simulink model "Copy_of_Formation_Controller"  (R2022b)
settings: Solver=VariableStepAuto  StartTime=0.0  StopTime=10.0  FixedStep=CONTROL_CONST.dt  MaxStep=0.01  RelTol=1e-3
values from neighbouring files (symbols this model uses):
  CONTROL_PARAM = Simulink.Parameter(CONTROL_PARAM_VALUE)    [control_model_init.m]
undefined symbols (not defined in the file or in its folder): actuator_cmd, CONTROL_CONST, CONTROL_PARAM_VALUE, CTRL_PARAM, DiscIntNeverNeededParam, FROMATION_PARAM, timestamp
libraries: FC_Lib x5, simulink x4, simulink_extras x1, aerolibasang x1
settings Model: VariantFading=off  Creator=19114  LastModifiedBy=19114
settings OptimizationCC: DefaultParameterBehavior=Inlined  DefaultUnderspecifiedDataType=single  EnhancedBackFolding=on  PassReuseOutputArgsAs=Individual arguments  ZeroExternalMemoryAtStartup=off  ZeroInternalMemoryAtStartup=off  OptimizeBlockOrder=speed  DifferentSizesBufferReuse=on  OptimizationCustomize=off  EfficientTunableParamExpr=on
settings DebuggingCC: ParameterTunabilityLossMsg=error
settings HardwareCC: ProdBitPerPointer=32  ProdBitPerSizeT=32  ProdBitPerPtrDiffT=32  ProdWordSize=32  ProdHWDeviceType=Intel->x86-32 (Windows32)
settings SFSimCC: MATLABDynamicMemAlloc=off
settings RTWCC: Description=Embedded Coder  SystemTargetFile=ert.tlc  TemplateMakefile=ert_default_tmf
settings CodeAppCC: ForceParamTrailComments=on  IgnoreCustomStorageClasses=off  OperatorAnnotations=on  SimulinkDataObjDesc=on  SFDataObjDesc=on  InsertBlockDesc=on
settings ERTTargetCC: TargetLangStandard=C99 (ISO)  GenerateSampleERTMain=on  SupportVariableSizeSignals=on  InlinedParameterPlacement=NonHierarchical  ERTCustomFileTemplate=example_file_process.tlc

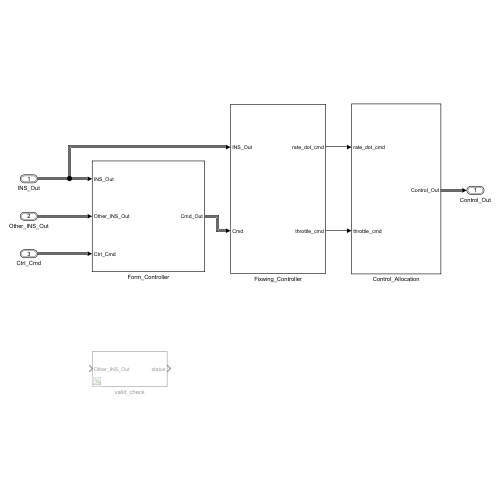
[thumbnail: Simulink's stored preview of the top-level diagram]
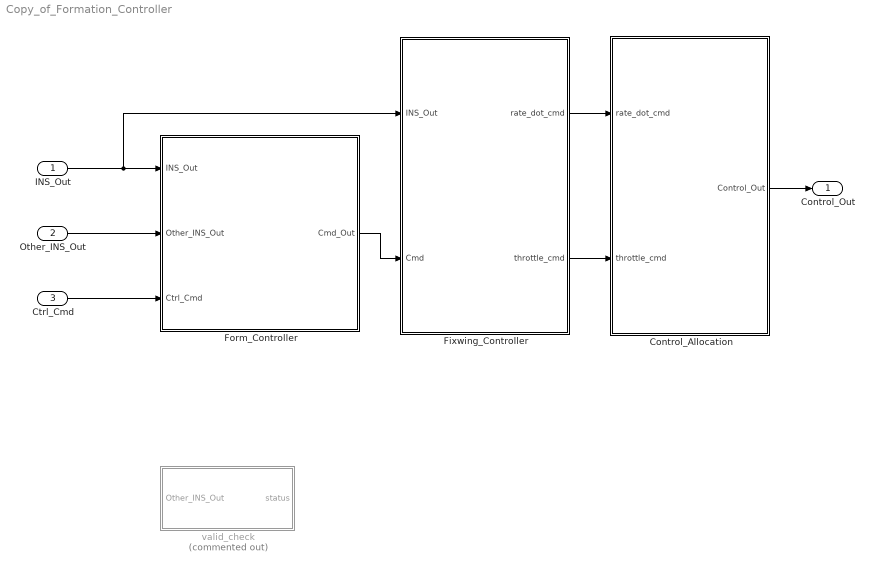
== system Copy_of_Formation_Controller ==
  INS_Out : Inport  OutDataTypeStr=Bus: INS_Out_Bus
  Other_INS_Out : Inport  Port=2  OutDataTypeStr=Bus: Other_INS_Out_Bus
  Ctrl_Cmd : Inport  Port=3  OutDataTypeStr=Bus: Cmd_In_Bus
  Control_Allocation : Subsystem
  Fixwing_Controller : Subsystem
  Form_Controller : Subsystem
  valid_check : Subsystem  Commented=on
  Control_Out : Outport  OutDataTypeStr=Bus: Control_Out_Bus
  wires:
  INS_Out/1 -> Fixwing_Controller/1(INS_Out), Form_Controller/1(INS_Out)
  Other_INS_Out/1 -> Form_Controller/2(Other_INS_Out)
  Ctrl_Cmd/1 -> Form_Controller/3(Ctrl_Cmd)
  Control_Allocation/1(Control_Out) -> Control_Out/1
  Form_Controller/1(Cmd_Out) -> Fixwing_Controller/2(Cmd)
  Fixwing_Controller/1(rate_dot_cmd) -> Control_Allocation/1(rate_dot_cmd)
  Fixwing_Controller/2(throttle_cmd) -> Control_Allocation/2(throttle_cmd)

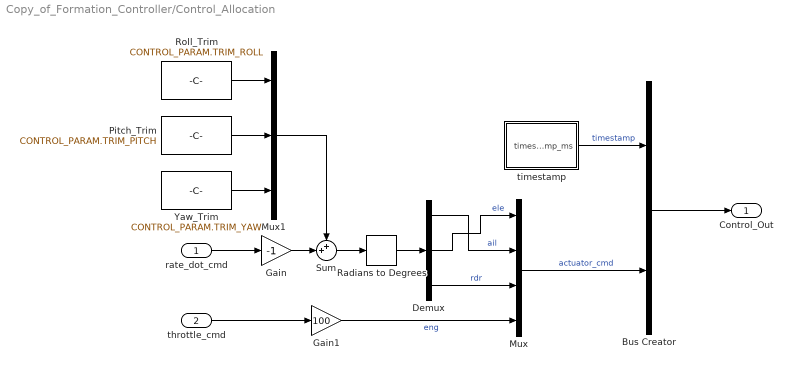
== system Copy_of_Formation_Controller/Control_Allocation ==
  rate_dot_cmd : Inport
  throttle_cmd : Inport  Port=2
  Bus Creator : BusCreator  Inputs=timestamp,actuator_cmd  OutDataTypeStr=Bus: Control_Out_Bus
  Demux : Demux  Outputs=3
  Gain : Gain  Gain=-1
  Gain1 : Gain  Gain=100
  Mux : Mux
  Mux1 : Mux  Inputs=3
  Pitch_Trim : Constant  Value=CONTROL_PARAM.TRIM_PITCH
  Radians to Degrees : simulink_extras/Transformations/Radians to Degrees
  Roll_Trim : Constant  Value=CONTROL_PARAM.TRIM_ROLL
  Sum : Sum  Inputs=++|
  Yaw_Trim : Constant  Value=CONTROL_PARAM.TRIM_YAW
  timestamp : Subsystem  mask{sample_time=CONTROL_CONST.dt*1000}
      mask prompts: sample_time "sample time (ms)"
  Control_Out : Outport
  wires:
  Bus Creator/1 -> Control_Out/1
  Mux/1 -> Bus Creator/2  "actuator_cmd"
  rate_dot_cmd/1 -> Gain/1
  throttle_cmd/1 -> Gain1/1
  Demux/1 -> Mux/2  "ail"
  Demux/2 -> Mux/1  "ele"
  Demux/3 -> Mux/3  "rdr"
  Sum/1 -> Radians to Degrees/1
  Mux1/1 -> Sum/1
  Gain/1 -> Sum/2
  Radians to Degrees/1 -> Demux/1
  Gain1/1 -> Mux/4  "eng"
  timestamp/1(timestamp_ms) -> Bus Creator/1  "timestamp"
  Roll_Trim/1 -> Mux1/1
  Pitch_Trim/1 -> Mux1/2
  Yaw_Trim/1 -> Mux1/3

== system Copy_of_Formation_Controller/Fixwing_Controller ==
  INS_Out : Inport
  Cmd : Inport  Port=2
  Attitude_Control : Subsystem
  Lateral_Longitudinal_Control : Subsystem
  rate_dot_cmd : Outport
  throttle_cmd : Outport  Port=2
  wires:
  Cmd/1 -> Lateral_Longitudinal_Control/2(Cmd)
  Attitude_Control/1(rate_dot_cmd) -> rate_dot_cmd/1
  INS_Out/1 -> Attitude_Control/1(INS_Out), Lateral_Longitudinal_Control/1(INS_Out)
  Lateral_Longitudinal_Control/2(throttle_cmd) -> throttle_cmd/1
  Lateral_Longitudinal_Control/1(att_cmd) -> Attitude_Control/2(att_cmd)

== system Copy_of_Formation_Controller/Form_Controller ==
  INS_Out : Inport
  Other_INS_Out : Inport  Port=2
  Ctrl_Cmd : Inport  Port=3
  Add : Sum
  Add1 : Sum
  Add2 : Sum
  Bus Creator : BusCreator  Inputs=3
  Consensus_Controller : Subsystem
  Local_State_Controller : Subsystem
  Cmd_Out : Outport
  wires:
  Add/1 -> Bus Creator/1  "cmd_ax"
  Local_State_Controller/1(ax_cmd) -> Add/1
  Consensus_Controller/1(ax_cmd) -> Add/2
  Add1/1 -> Bus Creator/2  "cmd_ay"
  Local_State_Controller/2(ay_cmd) -> Add1/1
  Local_State_Controller/3(vh_cmd) -> Add2/1
  Consensus_Controller/2(ay_cmd) -> Add1/2
  Add2/1 -> Bus Creator/3  "cmd_vh"
  Consensus_Controller/3(vh_cmd) -> Add2/2
  Other_INS_Out/1 -> Consensus_Controller/2(Other_INS_Out)
  Ctrl_Cmd/1 -> Local_State_Controller/1(Ctrl_Cmd)
  INS_Out/1 -> Consensus_Controller/1(INS_Out), Local_State_Controller/2(INS_Out)
  Bus Creator/1 -> Cmd_Out/1

== system Copy_of_Formation_Controller/valid_check ==
  Other_INS_Out : Inport
  Bus Selector1 : BusSelector  OutputSignals=timestamp
  Data Type Conversion : DataTypeConversion  OutDataTypeStr=uint32  SaturateOnIntegerOverflow=off  RndMeth=Floor
  Detect Increase : simulink/Logic and Bit Operations/Detect Increase  vinit=0.0  OutDataTypeStr=boolean
  Selector : Selector  InputPortWidth=20  IndexOptions=Index vector (dialog)  Indices=[1:CTRL_PARAM.NUM_UAV]  OutputSizes=1
  status : Outport
  wires:
  Other_INS_Out/1 -> Bus Selector1/1
  Detect Increase/1 -> Selector/1
  Bus Selector1/1 -> Detect Increase/1  "<timestamp>"
  Selector/1 -> Data Type Conversion/1
  Data Type Conversion/1 -> status/1  "status"

== system Copy_of_Formation_Controller/Control_Allocation/timestamp ==
  Add : Sum
  Constant : Constant  Value=sample_time  OutDataTypeStr=uint32
  Memory : Memory
  timestamp_ms : Outport  VectorParamsAs1DForOutWhenUnconnected=off
  wires:
  Constant/1 -> Add/1
  Add/1 -> Memory/1, timestamp_ms/1
  Memory/1 -> Add/2

== system Copy_of_Formation_Controller/Fixwing_Controller/Attitude_Control ==
  INS_Out : Inport
  att_cmd : Inport  Port=2
  Innerloop_Rate_Control : Subsystem
  Outloop_Angle_Control : Subsystem
  rate_dot_cmd : Outport  VectorParamsAs1DForOutWhenUnconnected=off
  wires:
  Outloop_Angle_Control/1(euler_rate_cmd) -> Innerloop_Rate_Control/1(euler_rate_cmd)
  INS_Out/1 -> Innerloop_Rate_Control/2(INS_Out), Outloop_Angle_Control/2(INS_Out)
  Innerloop_Rate_Control/1(rate_dot_cmd) -> rate_dot_cmd/1
  att_cmd/1 -> Outloop_Angle_Control/1(att_cmd)

== system Copy_of_Formation_Controller/Fixwing_Controller/Lateral_Longitudinal_Control ==
  INS_Out : Inport
  Cmd : Inport  Port=2
  Airspeed_Filter : Subsystem
  Altitude_Control : Subsystem
  Lateral_Control : Subsystem
  Longitudinal_Control : Subsystem
  Mux : Mux  Inputs=2
  att_cmd : Outport  VectorParamsAs1DForOutWhenUnconnected=off
  throttle_cmd : Outport  Port=2  VectorParamsAs1DForOutWhenUnconnected=off
  wires:
  Cmd/1 -> Lateral_Control/1(Cmd), Airspeed_Filter/1(Cmd), Altitude_Control/1(Cmd)
  Altitude_Control/1(alt_rate_sp) -> Longitudinal_Control/1(alt_rate_sp)
  INS_Out/1 -> Longitudinal_Control/4(INS_Out), Airspeed_Filter/2(INS_Out), Altitude_Control/2(INS_Out)
  Longitudinal_Control/1(pitch_cmd) -> Mux/2  "pitch_cmd"
  Altitude_Control/2(alt_rate) -> Longitudinal_Control/2(alt_rate)
  Longitudinal_Control/2(throttle_cmd) -> throttle_cmd/1
  Airspeed_Filter/1(airspeed) -> Longitudinal_Control/3(airspeed)
  Lateral_Control/1(roll_cmd) -> Mux/1  "roll_cmd"
  Mux/1 -> att_cmd/1

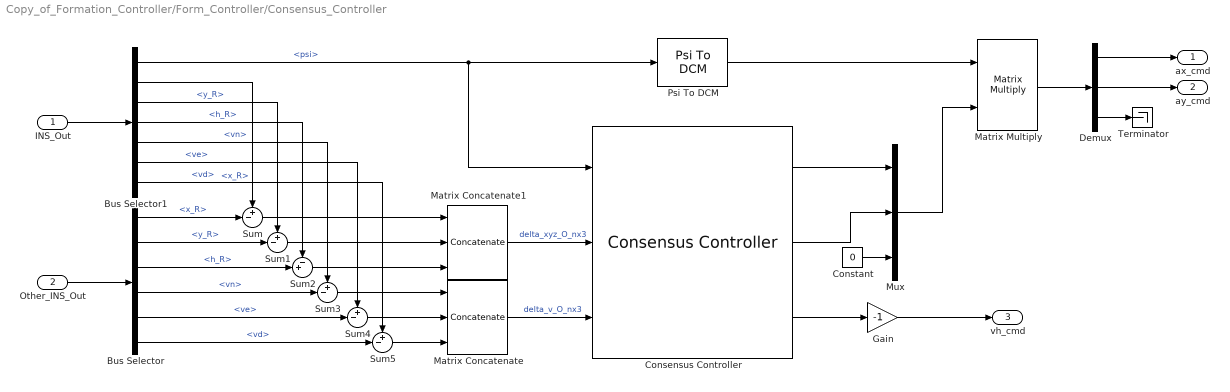
== system Copy_of_Formation_Controller/Form_Controller/Consensus_Controller ==
  INS_Out : Inport
  Other_INS_Out : Inport  Port=2
  Bus Selector : BusSelector  OutputSignals=x_R,y_R,h_R,vn,ve,vd
  Bus Selector1 : BusSelector  OutputSignals=psi,x_R,y_R,h_R,vn,ve,vd
  Consensus Controller : FC_Lib/Fromation/Consensus Controller  uav_id=FROMATION_PARAM.UAV_ID+1  adj_matrix=FROMATION_PARAM.ADJ_MARTIX  rel_x=FROMATION_PARAM.REL_X_MATRIX  rel_y=FROMATION_PARAM.REL_Y_MATRIX  rel_z=FROMATION_PARAM.REL_Z_MATRIX  kx=FROMATION_PARAM.FORM_X_KP  ky=FROMATION_PARAM.FORM_Y_KP  kz=FROMATION_PARAM.FORM_Z_KP
      settings: LibrarySourceBlock=|
      | simulink/User-Defined
      | Functions/MATLAB Function
  Constant : Constant  Value=0  OutDataTypeStr=single
  Demux : Demux  Outputs=3
  Gain : Gain  Gain=-1
  Matrix Concatenate : Concatenate  NumInputs=3  Mode=Multidimensional array  ConcatenateDimension=2
  Matrix Concatenate1 : Concatenate  NumInputs=3  Mode=Multidimensional array  ConcatenateDimension=2
  Matrix Multiply : Product  Multiplication=Matrix(*)
  Mux : Mux  Inputs=3
  Psi To DCM : FC_Lib/Transformation/Psi To DCM
      settings: SourceProductName=Flight Control Toolbox
  Sum{,1,3..5} (5 alike) : Sum  Inputs=+-|
  Sum2 : Sum  Inputs=-+|
  Terminator : Terminator
  ax_cmd : Outport
  ay_cmd : Outport  Port=2
  vh_cmd : Outport  Port=3
  wires:
  Bus Selector1/4 -> Sum2/1  "<h_R>"
  Bus Selector/6 -> Sum5/2  "<vd>"
  Other_INS_Out/1 -> Bus Selector/1
  Bus Selector/2 -> Sum1/2  "<y_R>"
  Sum2/1 -> Matrix Concatenate1/3
  INS_Out/1 -> Bus Selector1/1
  Bus Selector/5 -> Sum4/2  "<ve>"
  Bus Selector1/7 -> Sum5/1  "<vd>"
  Bus Selector1/6 -> Sum4/1  "<ve>"
  Bus Selector1/2 -> Sum/1  "<x_R>"
  Bus Selector/3 -> Sum2/2  "<h_R>"
  Bus Selector/1 -> Sum/2  "<x_R>"
  Bus Selector/4 -> Sum3/2  "<vn>"
  Sum4/1 -> Matrix Concatenate/2
  Sum1/1 -> Matrix Concatenate1/2
  Bus Selector1/5 -> Sum3/1  "<vn>"
  Sum5/1 -> Matrix Concatenate/3
  Matrix Concatenate/1 -> Consensus Controller/3  "delta_v_O_nx3"
  Sum/1 -> Matrix Concatenate1/1
  Matrix Concatenate1/1 -> Consensus Controller/2  "delta_xyz_O_nx3"
  Bus Selector1/3 -> Sum1/1  "<y_R>"
  Consensus Controller/3 -> Gain/1
  Sum3/1 -> Matrix Concatenate/1
  Consensus Controller/2 -> Mux/2
  Consensus Controller/1 -> Mux/1
  Gain/1 -> vh_cmd/1
  Constant/1 -> Mux/3
  Psi To DCM/1 -> Matrix Multiply/1
  Mux/1 -> Matrix Multiply/2
  Matrix Multiply/1 -> Demux/1
  Demux/3 -> Terminator/1
  Bus Selector1/1 -> Consensus Controller/1, Psi To DCM/1  "<psi>"
  Demux/1 -> ax_cmd/1
  Demux/2 -> ay_cmd/1

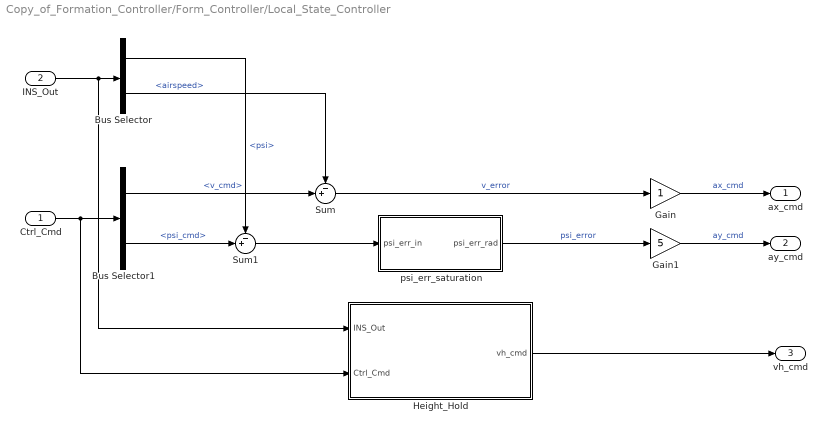
== system Copy_of_Formation_Controller/Form_Controller/Local_State_Controller ==
  Ctrl_Cmd : Inport
  INS_Out : Inport  Port=2
  Bus Selector : BusSelector  OutputSignals=psi,airspeed
  Bus Selector1 : BusSelector  OutputSignals=v_cmd,psi_cmd
  Gain : Gain
  Gain1 : Gain  Gain=5
  Height_Hold : Subsystem
  Sum : Sum  Inputs=-+|
  Sum1 : Sum  Inputs=-+|
  psi_err_saturation : Subsystem
  ax_cmd : Outport
  ay_cmd : Outport  Port=2
  vh_cmd : Outport  Port=3
  wires:
  Sum/1 -> Gain/1  "v_error"
  Sum1/1 -> psi_err_saturation/1(psi_err_in)
  Gain/1 -> ax_cmd/1  "ax_cmd"
  Gain1/1 -> ay_cmd/1  "ay_cmd"
  Bus Selector/1 -> Sum1/1  "<psi>"
  Bus Selector1/1 -> Sum/2  "<v_cmd>"
  Bus Selector1/2 -> Sum1/2  "<psi_cmd>"
  psi_err_saturation/1(psi_err_rad) -> Gain1/1  "psi_error"
  Ctrl_Cmd/1 -> Height_Hold/2(Ctrl_Cmd), Bus Selector1/1
  INS_Out/1 -> Height_Hold/1(INS_Out), Bus Selector/1
  Height_Hold/1(vh_cmd) -> vh_cmd/1
  Bus Selector/2 -> Sum/1  "<airspeed>"

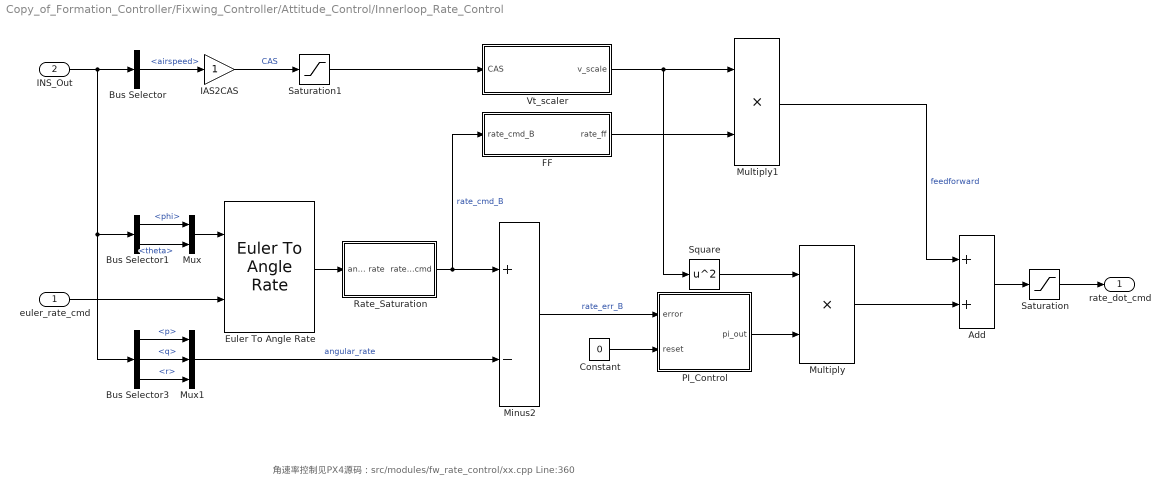
== system Copy_of_Formation_Controller/Fixwing_Controller/Attitude_Control/Innerloop_Rate_Control ==
  note: 角速率控制见PX4源码：src/modules/fw_rate_control/xx.cpp Line:360
  euler_rate_cmd : Inport
  INS_Out : Inport  Port=2
  Add : Sum
  Bus Selector : BusSelector  OutputSignals=airspeed
  Bus Selector1 : BusSelector  OutputSignals=phi,theta
  Bus Selector3 : BusSelector  OutputSignals=p,q,r
  Constant : Constant  Value=0
  Euler To Angle Rate : FC_Lib/Math/Euler To Angle Rate
      settings: SourceProductName=Flight Control Toolbox
  FF : Subsystem
  IAS2CAS : Gain
  Minus2 : Sum  Inputs=+-
  Multiply : Product
  Multiply1 : Product
  Mux : Mux  Inputs=2
  Mux1 : Mux  Inputs=3
  PI_Control : Subsystem
  Rate_Saturation : Subsystem
  Saturation : Saturate  UpperLimit=1  LowerLimit=-1
  Saturation1 : Saturate  UpperLimit=inf  LowerLimit=0.5
  Square : Math  Operator=square
  Vt_scaler : Subsystem
  rate_dot_cmd : Outport  VectorParamsAs1DForOutWhenUnconnected=off
  wires:
  Vt_scaler/1(v_scale) -> Square/1, Multiply1/1
  FF/1(rate_ff) -> Multiply1/2
  Multiply1/1 -> Add/1  "feedforward"
  Bus Selector/1 -> IAS2CAS/1  "<airspeed>"
  euler_rate_cmd/1 -> Euler To Angle Rate/2
  Euler To Angle Rate/1 -> Rate_Saturation/1(angle rate)
  Mux1/1 -> Minus2/2  "angular_rate"
  Add/1 -> Saturation/1
  Minus2/1 -> PI_Control/1(error)  "rate_err_B"
  PI_Control/1(pi_out) -> Multiply/2
  INS_Out/1 -> Bus Selector/1, Bus Selector3/1, Bus Selector1/1
  Bus Selector1/1 -> Mux/1  "<phi>"
  Bus Selector1/2 -> Mux/2  "<theta>"
  Mux/1 -> Euler To Angle Rate/1
  Bus Selector3/1 -> Mux1/1  "<p>"
  Bus Selector3/2 -> Mux1/2  "<q>"
  Bus Selector3/3 -> Mux1/3  "<r>"
  Saturation1/1 -> Vt_scaler/1(CAS)
  IAS2CAS/1 -> Saturation1/1  "CAS"
  Square/1 -> Multiply/1
  Saturation/1 -> rate_dot_cmd/1
  Constant/1 -> PI_Control/2(reset)
  Multiply/1 -> Add/2
  Rate_Saturation/1(rate_cmd) -> FF/1(rate_cmd_B), Minus2/1  "rate_cmd_B"

== system Copy_of_Formation_Controller/Fixwing_Controller/Attitude_Control/Outloop_Angle_Control ==
  att_cmd : Inport
  INS_Out : Inport  Port=2
  Attitude_Controller : Subsystem
  Heading_Controller : Subsystem
  Mux : Mux  Inputs=2
  Reshape : Reshape  OutputDimensionality=Column vector (2-D)
  euler_rate_cmd : Outport  VectorParamsAs1DForOutWhenUnconnected=off
  wires:
  INS_Out/1 -> Heading_Controller/2(INS_Out), Attitude_Controller/2(INS_Out)
  Attitude_Controller/1(phi_theta_rate_cmd) -> Mux/1
  Heading_Controller/1(psi_rate_cmd) -> Mux/2
  Mux/1 -> Reshape/1
  Reshape/1 -> euler_rate_cmd/1
  att_cmd/1 -> Heading_Controller/1(att_cmd), Attitude_Controller/1(att_cmd)

== system Copy_of_Formation_Controller/Fixwing_Controller/Lateral_Longitudinal_Control/Airspeed_Filter ==
  Cmd : Inport
  INS_Out : Inport  Port=2
  Bus Creator : BusCreator  Inputs=3
  Bus Selector1 : BusSelector  OutputSignals=airspeed
  Calc_TAS_Rate_Setpoint : Subsystem
  Constant : Constant  Value=0  OutDataTypeStr=single
  Ideal Airspeed Correction : aerolibasang/Ideal Airspeed Correction  Commented=on  units=Metric (MKS)  vel_in=CAS  vel_out_tas=CAS  vel_out_eas=TAS  vel_out_cas=TAS  method=Table Lookup  SubOnly=on  action=None
  Saturation2 : Saturate  UpperLimit=inf  LowerLimit=0
  Second Order DT Filter : FC_Lib/Filter/Second Order DT Filter  fc=10  zeta=1
      settings: SourceProductName=Flight Control Toolbox
  airspeed : Outport
  wires:
  INS_Out/1 -> Bus Selector1/1
  Bus Creator/1 -> airspeed/1
  Bus Selector1/1 -> Second Order DT Filter/1, Saturation2/1, Calc_TAS_Rate_Setpoint/2(TAS_mPs)  "<airspeed>"
  Cmd/1 -> Calc_TAS_Rate_Setpoint/1(Cmd)
  Calc_TAS_Rate_Setpoint/1(TAS_rate_sp_mPs) -> Bus Creator/1  "TAS_rate_sp_mPs"
  Saturation2/1 -> Bus Creator/2  "TAS_mPs"
  Second Order DT Filter/1 -> Bus Creator/3  "TAS_rate_mPs"
  Constant/1 -> Second Order DT Filter/2

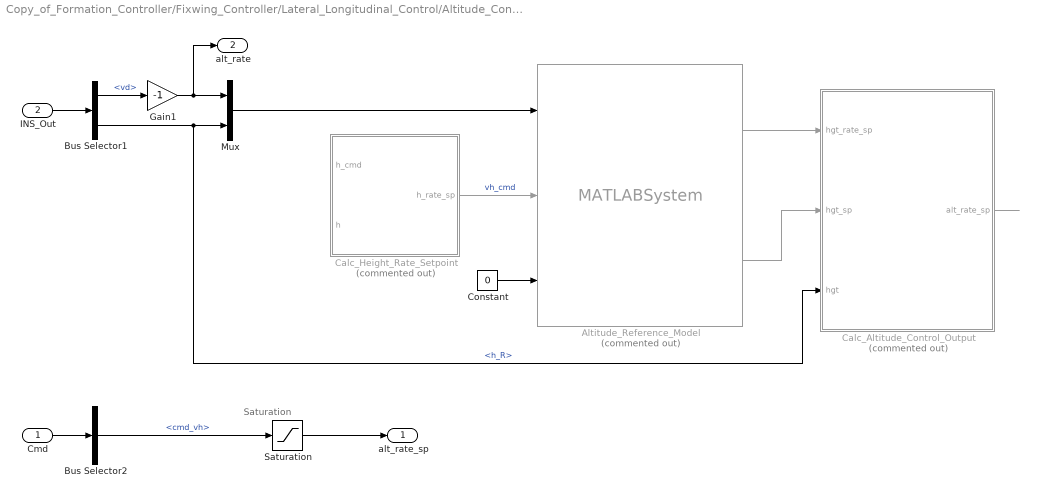
== system Copy_of_Formation_Controller/Fixwing_Controller/Lateral_Longitudinal_Control/Altitude_Control ==
  note: Saturation
  Cmd : Inport
  INS_Out : Inport  Port=2
  Altitude_Reference_Model : MATLABSystem  Commented=on  System=VelocitySmoothing  max_jerk=single(1000)  max_accel=CONTROL_PARAM.FW_T_VERT_ACC  max_climb_rate=CONTROL_PARAM.FW_T_CLMB_MAX  max_sink_rate=CONTROL_PARAM.FW_T_SINK_MAX  SampleTime=CONTROL_CONST.dt  SimulateUsing=Code generation
      mask Type: VelocitySmoothing
      mask Display:
      | disp(['Velocity' char(10) 'Smoothing']);
      | port_label('input',1,'v0x0');
      | port_label('input',2,'vel_sp');
      | port_label('input',3,'reset');
      | port_label('output',1,'vel');
      | port_label('output',2,'pos');
  Bus Selector1 : BusSelector  OutputSignals=vd,h_R
  Bus Selector2 : BusSelector  OutputSignals=cmd_vh
  Calc_Altitude_Control_Output : Subsystem  Commented=on
  Calc_Height_Rate_Setpoint : Subsystem  Commented=on
  Constant : Constant  Value=0  OutDataTypeStr=single
  Gain1 : Gain  Gain=-1
  Mux : Mux  Inputs=2
  Saturation : Saturate  UpperLimit=CONTROL_PARAM.FW_T_CLMB_MAX  LowerLimit=-CONTROL_PARAM.FW_T_SINK_MAX
  alt_rate_sp : Outport
  alt_rate : Outport  Port=2
  wires:
  Cmd/1 -> Bus Selector2/1
  INS_Out/1 -> Bus Selector1/1
  Bus Selector1/2 -> Mux/2, Calc_Altitude_Control_Output/3(hgt)  "<h_R>"
  Bus Selector2/1 -> Saturation/1  "<cmd_vh>"
  Bus Selector1/1 -> Gain1/1  "<vd>"
  Gain1/1 -> Mux/1, alt_rate/1
  Mux/1 -> Altitude_Reference_Model/1
  Altitude_Reference_Model/2 -> Calc_Altitude_Control_Output/2(hgt_sp)
  Constant/1 -> Altitude_Reference_Model/3
  Altitude_Reference_Model/1 -> Calc_Altitude_Control_Output/1(hgt_rate_sp)
  Calc_Altitude_Control_Output/1(alt_rate_sp) -> ?
  Calc_Height_Rate_Setpoint/1(h_rate_sp) -> Altitude_Reference_Model/2  "vh_cmd"
  Saturation/1 -> alt_rate_sp/1

== system Copy_of_Formation_Controller/Fixwing_Controller/Lateral_Longitudinal_Control/Lateral_Control ==
  Cmd : Inport
  Atan : Trigonometry  Operator=atan
  Bus Selector : BusSelector  OutputSignals=cmd_ay
  Constant : Constant  Value=CONTROL_CONST.g
  Product : Product  Inputs=/*
  Saturation : Saturate  UpperLimit=CONTROL_PARAM.FW_R_LIM  LowerLimit=-CONTROL_PARAM.FW_R_LIM
  roll_cmd : Outport
  wires:
  Cmd/1 -> Bus Selector/1
  Constant/1 -> Product/1
  Bus Selector/1 -> Product/2  "<cmd_ay>"
  Product/1 -> Atan/1
  Atan/1 -> Saturation/1
  Saturation/1 -> roll_cmd/1

== system Copy_of_Formation_Controller/Fixwing_Controller/Lateral_Longitudinal_Control/Longitudinal_Control ==
  alt_rate_sp : Inport
  alt_rate : Inport  Port=2
  airspeed : Inport  Port=3
  INS_Out : Inport  Port=4
  Bus Selector : BusSelector  OutputSignals=TAS_mPs
  Calc_Specific_Energy_Rates : Subsystem
  Pitch_Control : Subsystem
  Throttle_Control : Subsystem
  pitch_cmd : Outport
  throttle_cmd : Outport  Port=2
  wires:
  alt_rate_sp/1 -> Calc_Specific_Energy_Rates/1(alt_rate_sp)
  alt_rate/1 -> Calc_Specific_Energy_Rates/2(alt_rate)
  Throttle_Control/1(throttle_cmd) -> throttle_cmd/1
  Pitch_Control/1(pitch_cmd) -> pitch_cmd/1
  INS_Out/1 -> Throttle_Control/2(INS_Out)
  Calc_Specific_Energy_Rates/1(ser) -> Pitch_Control/1(ser), Throttle_Control/1(ser)
  Bus Selector/1 -> Pitch_Control/2(tas)  "<TAS_mPs>"
  airspeed/1 -> Bus Selector/1, Calc_Specific_Energy_Rates/3(airspeed)

== system Copy_of_Formation_Controller/Form_Controller/Local_State_Controller/Height_Hold ==
  INS_Out : Inport
  Ctrl_Cmd : Inport  Port=2
  Bus Selector2 : BusSelector  OutputSignals=h_cmd
  Bus Selector3 : BusSelector  OutputSignals=h_R
  Gain3 : Gain
  Sum3 : Sum  Inputs=-+|
  vh_cmd : Outport
  wires:
  Bus Selector3/1 -> Sum3/1  "<h_R>"
  Sum3/1 -> Gain3/1  "h_error"
  INS_Out/1 -> Bus Selector3/1
  Bus Selector2/1 -> Sum3/2  "<h_cmd>"
  Ctrl_Cmd/1 -> Bus Selector2/1
  Gain3/1 -> vh_cmd/1

== system Copy_of_Formation_Controller/Form_Controller/Local_State_Controller/psi_err_saturation ==
  psi_err_in : Inport
  Abs : Abs  SaturateOnIntegerOverflow=off
  Compare To Constant : simulink/Logic and Bit Operations/Compare To Constant  relop=>  const=pi  OutDataTypeStr=boolean
  Constant : Constant  Value=2*pi  OutDataTypeStr=single
  Multiply : Product
  Sign : Signum
  Subtract : Sum  Inputs=-+
  Switch : Switch  Criteria=u2 > Threshold  SaturateOnIntegerOverflow=off  InputSameDT=off
  psi_err_rad : Outport  VectorParamsAs1DForOutWhenUnconnected=off
  wires:
  Multiply/1 -> Switch/1
  Sign/1 -> Multiply/2
  Subtract/1 -> Multiply/1
  Constant/1 -> Subtract/1
  Switch/1 -> psi_err_rad/1
  Compare To Constant/1 -> Switch/2
  Abs/1 -> Compare To Constant/1, Subtract/2
  psi_err_in/1 -> Abs/1, Switch/3, Sign/1

== system Copy_of_Formation_Controller/Fixwing_Controller/Attitude_Control/Innerloop_Rate_Control/FF ==
  rate_cmd_B : Inport
  Demux : Demux  Outputs=3
  Mux2 : Mux  Inputs=3
  pitch_ff : Gain  Gain=CONTROL_PARAM.FW_PR_FF
  roll_ff : Gain  Gain=CONTROL_PARAM.FW_RR_FF
  yaw_ff : Gain  Gain=CONTROL_PARAM.FW_YR_FF
  rate_ff : Outport
  wires:
  Mux2/1 -> rate_ff/1
  Demux/2 -> pitch_ff/1  "pitch_rate"
  Demux/1 -> roll_ff/1  "roll_rate"
  Demux/3 -> yaw_ff/1  "yaw_rate"
  rate_cmd_B/1 -> Demux/1
  roll_ff/1 -> Mux2/1
  pitch_ff/1 -> Mux2/2
  yaw_ff/1 -> Mux2/3

== system Copy_of_Formation_Controller/Fixwing_Controller/Attitude_Control/Innerloop_Rate_Control/PI_Control ==
  error : Inport
  reset : Inport  Port=2
  Add1 : Sum
  I_Control : Subsystem  mask{p_ki=CONTROL_PARAM.ROLL_RATE_I, q_ki=CONTROL_PARAM.PITCH_RATE_I, r_ki=CONTROL_PARAM.YAW_RATE_I, max_i=CONTROL_PARAM.RATE_I_MAX, min_i=CONTROL_PARAM.RATE_I_MIN}
  P_Control : Subsystem  mask{p_kp=CONTROL_PARAM.ROLL_RATE_P, q_kp=CONTROL_PARAM.PITCH_RATE_P, r_kp=CONTROL_PARAM.YAW_RATE_P}
  pi_out : Outport  VectorParamsAs1DForOutWhenUnconnected=off
  wires:
  Add1/1 -> pi_out/1
  I_Control/1(i_out) -> Add1/2  "i_out"
  error/1 -> P_Control/1(err), I_Control/1(err)
  P_Control/1(p_out) -> Add1/1
  reset/1 -> I_Control/2(reset)

== system Copy_of_Formation_Controller/Fixwing_Controller/Attitude_Control/Innerloop_Rate_Control/Rate_Saturation ==
  angle rate : Inport
  Demux : Demux  Outputs=3
  Mux : Mux  Inputs=3
  Saturation : Saturate  UpperLimit=CONTROL_PARAM.FW_R_RMAX  LowerLimit=-CONTROL_PARAM.FW_R_RMAX
  Saturation1 : Saturate  UpperLimit=CONTROL_PARAM.FW_P_RMAX  LowerLimit=-CONTROL_PARAM.FW_P_RMAX
  Saturation2 : Saturate  UpperLimit=CONTROL_PARAM.FW_Y_RMAX  LowerLimit=-CONTROL_PARAM.FW_Y_RMAX
  rate_cmd : Outport
  wires:
  angle rate/1 -> Demux/1
  Mux/1 -> rate_cmd/1
  Demux/1 -> Saturation/1  "roll_rate"
  Demux/2 -> Saturation1/1  "pitch_rate"
  Demux/3 -> Saturation2/1  "yaw_rate"
  Saturation/1 -> Mux/1
  Saturation1/1 -> Mux/2
  Saturation2/1 -> Mux/3

== system Copy_of_Formation_Controller/Fixwing_Controller/Attitude_Control/Innerloop_Rate_Control/Vt_scaler ==
  CAS : Inport
  CAS_constrained : Saturate  UpperLimit=CONTROL_PARAM.FW_AIRSPD_MAX  LowerLimit=CONTROL_PARAM.FW_AIRSPD_STALL
  Constant1 : Constant  Value=CONTROL_PARAM.FW_ARSP_SCALE_EN
  Constant2 : Constant  OutDataTypeStr=single
  Divide : Product  Inputs=/*
  Switch1 : Switch  Criteria=u2 > Threshold  SaturateOnIntegerOverflow=off  InputSameDT=off
  Trim_CAS : Constant  Value=CONTROL_PARAM.FW_AIRSPD_TRIM
  v_scale : Outport
  wires:
  CAS_constrained/1 -> Divide/1
  Divide/1 -> Switch1/1
  Constant1/1 -> Switch1/2
  Switch1/1 -> v_scale/1
  Trim_CAS/1 -> Divide/2
  Constant2/1 -> Switch1/3
  CAS/1 -> CAS_constrained/1

== system Copy_of_Formation_Controller/Fixwing_Controller/Attitude_Control/Outloop_Angle_Control/Attitude_Controller ==
  att_cmd : Inport
  INS_Out : Inport  Port=2
  Error : Subsystem
  P_Controller : Subsystem
  phi_theta_rate_cmd : Outport  VectorParamsAs1DForOutWhenUnconnected=off
  wires:
  INS_Out/1 -> Error/2(INS_Out)
  P_Controller/1(u) -> phi_theta_rate_cmd/1
  att_cmd/1 -> Error/1(att_cmd)
  Error/1(euler_err_rad) -> P_Controller/1(error)

== system Copy_of_Formation_Controller/Fixwing_Controller/Attitude_Control/Outloop_Angle_Control/Heading_Controller ==
  att_cmd : Inport
  INS_Out : Inport  Port=2
  Selector : Selector  InputPortWidth=2  IndexOptions=Index vector (dialog)  Indices=[1]  OutputSizes=1
  Turning_Coordination : Subsystem
  psi_rate_cmd : Outport  VectorParamsAs1DForOutWhenUnconnected=off
  wires:
  Turning_Coordination/1(psi_rate_sp) -> psi_rate_cmd/1
  INS_Out/1 -> Turning_Coordination/2(INS_Out)
  att_cmd/1 -> Selector/1
  Selector/1 -> Turning_Coordination/1(phi_sp)

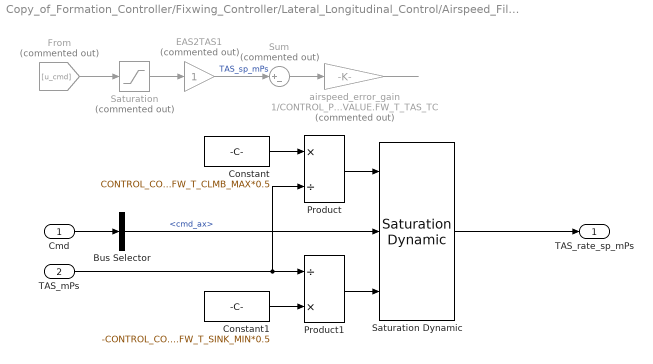
== system Copy_of_Formation_Controller/Fixwing_Controller/Lateral_Longitudinal_Control/Airspeed_Filter/Calc_TAS_Rate_Setpoint ==
  Cmd : Inport
  TAS_mPs : Inport  Port=2
  Bus Selector : BusSelector  OutputSignals=cmd_ax
  Constant : Constant  Value=CONTROL_CONST.g*CONTROL_PARAM.FW_T_CLMB_MAX*0.5  OutDataTypeStr=single
  Constant1 : Constant  Value=-CONTROL_CONST.g*CONTROL_PARAM.FW_T_SINK_MIN*0.5  OutDataTypeStr=single
  EAS2TAS1 : Gain  Commented=on
  From : From  Commented=on  GotoTag=u_cmd
  Product : Product  Inputs=*/
  Product1 : Product  Inputs=/*
  Saturation : Saturate  Commented=on  UpperLimit=CONTROL_PARAM.FW_AIRSPD_MAX  LowerLimit=CONTROL_PARAM.FW_AIRSPD_MIN
  Saturation Dynamic : simulink/Discontinuities/Saturation Dynamic  OutMin=[]  OutMax=[]  OutDataTypeStr=Inherit: Same as second input  OutDataType=fixdt(1, 16)  OutScaling=2^-10  DoSatur=off
  Sum : Sum  Commented=on  Inputs=|+-
  airspeed_error_gain : Gain  Commented=on  Gain=1/CONTROL_PARAM_VALUE.FW_T_TAS_TC
  TAS_rate_sp_mPs : Outport
  wires:
  Saturation Dynamic/1 -> TAS_rate_sp_mPs/1
  Sum/1 -> airspeed_error_gain/1
  Cmd/1 -> Bus Selector/1
  TAS_mPs/1 -> Product/2, Product1/1
  airspeed_error_gain/1 -> ?
  Constant/1 -> Product/1
  Product/1 -> Saturation Dynamic/1
  Product1/1 -> Saturation Dynamic/3
  Constant1/1 -> Product1/2
  From/1 -> Saturation/1
  EAS2TAS1/1 -> Sum/1  "TAS_sp_mPs"
  Saturation/1 -> EAS2TAS1/1
  Bus Selector/1 -> Saturation Dynamic/2  "<cmd_ax>"

== system Copy_of_Formation_Controller/Fixwing_Controller/Lateral_Longitudinal_Control/Altitude_Control/Calc_Altitude_Control_Output ==
  note: Saturation
  hgt_rate_sp : Inport
  hgt_sp : Inport  Port=2
  hgt : Inport  Port=3
  Gain : Gain  Gain=CONTROL_PARAM.FW_T_HRATE_FF
  Gain2 : Gain  Gain=1/max(CONTROL_PARAM.FW_T_ALT_TC,0.1)
  Saturation : Saturate  UpperLimit=CONTROL_PARAM.FW_T_CLMB_MAX  LowerLimit=-CONTROL_PARAM.FW_T_SINK_MAX
  Sum : Sum  Inputs=|++
  Sum1 : Sum  Inputs=|+-
  alt_rate_sp : Outport
  wires:
  Sum1/1 -> Gain2/1
  hgt_sp/1 -> Sum1/1
  Gain/1 -> Sum/1  "alt_rate_gain_ff"
  hgt_rate_sp/1 -> Gain/1
  hgt/1 -> Sum1/2
  Sum/1 -> Saturation/1
  Gain2/1 -> Sum/2  "alt_gain"
  Saturation/1 -> alt_rate_sp/1

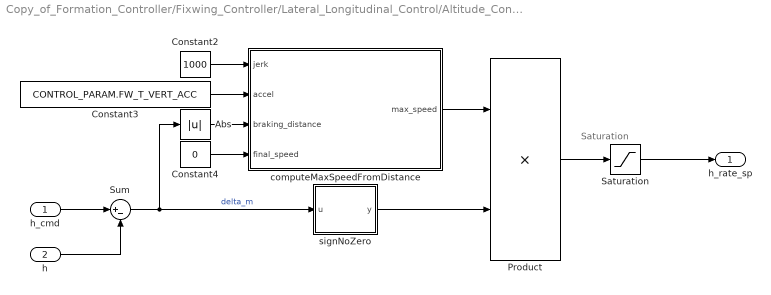
== system Copy_of_Formation_Controller/Fixwing_Controller/Lateral_Longitudinal_Control/Altitude_Control/Calc_Height_Rate_Setpoint ==
  note: Saturation
  h_cmd : Inport
  h : Inport  Port=2
  Abs : Abs  SaturateOnIntegerOverflow=off
  Constant2 : Constant  Value=1000  OutDataTypeStr=single
  Constant3 : Constant  Value=CONTROL_PARAM.FW_T_VERT_ACC  OutDataTypeStr=single
  Constant4 : Constant  Value=0  OutDataTypeStr=single
  Product : Product
  Saturation : Saturate  UpperLimit=min(CONTROL_PARAM.FW_T_CLMB_R_SP, CONTROL_PARAM.FW_T_CLMB_MAX)  LowerLimit=-min(CONTROL_PARAM.FW_T_SINK_R_SP, CONTROL_PARAM.FW_T_SINK_MAX)
  Sum : Sum  Inputs=|+-  OutDataTypeStr=Inherit: Same as first input
  computeMaxSpeedFromDistance : MATLAB Function  TreatAsAtomicUnit=on
  signNoZero : MATLAB Function  TreatAsAtomicUnit=on
  h_rate_sp : Outport  OutDataTypeStr=single
  wires:
  computeMaxSpeedFromDistance/1(max_speed) -> Product/1
  Constant3/1 -> computeMaxSpeedFromDistance/2(accel)
  h/1 -> Sum/2
  Sum/1 -> Abs/1, signNoZero/1(u)  "delta_m"
  Abs/1 -> computeMaxSpeedFromDistance/3(braking_distance)
  Constant2/1 -> computeMaxSpeedFromDistance/1(jerk)
  Constant4/1 -> computeMaxSpeedFromDistance/4(final_speed)
  signNoZero/1(y) -> Product/2
  h_cmd/1 -> Sum/1
  Product/1 -> Saturation/1
  Saturation/1 -> h_rate_sp/1

== system Copy_of_Formation_Controller/Fixwing_Controller/Lateral_Longitudinal_Control/Longitudinal_Control/Calc_Specific_Energy_Rates ==
  alt_rate_sp : Inport
  alt_rate : Inport  Port=2
  airspeed : Inport  Port=3
  Bus Creator : BusCreator  Inputs=4
  Bus Selector : BusSelector  OutputSignals=TAS_mPs,TAS_rate_sp_mPs,TAS_rate_mPs
  Constant : Constant  Value=CONTROL_CONST.g
  Product{1..4} (4 alike) : Product
  ser : Outport
  wires:
  Product4/1 -> Bus Creator/1  "spe_rate_sp"
  airspeed/1 -> Bus Selector/1
  Bus Selector/1 -> Product3/2, Product1/1  "<TAS_mPs>"
  Bus Selector/2 -> Product1/2  "<TAS_rate_sp_mPs>"
  Product1/1 -> Bus Creator/3  "ske_rate_sp"
  Bus Selector/3 -> Product3/1  "<TAS_rate_mPs>"
  Product2/1 -> Bus Creator/2  "spe_rate"
  Product3/1 -> Bus Creator/4  "ske_rate"
  Bus Creator/1 -> ser/1
  Constant/1 -> Product4/2, Product2/1
  alt_rate/1 -> Product2/2
  alt_rate_sp/1 -> Product4/1

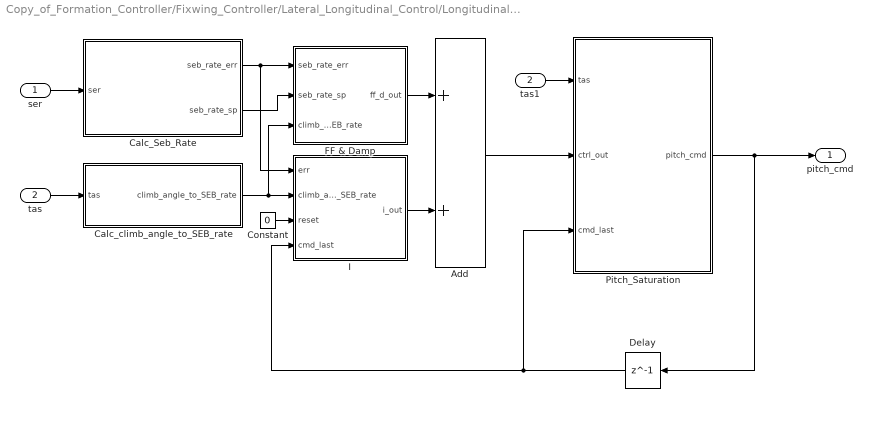
== system Copy_of_Formation_Controller/Fixwing_Controller/Lateral_Longitudinal_Control/Longitudinal_Control/Pitch_Control ==
  ser : Inport
  tas : Inport  Port=2
  Add : Sum
  Calc_Seb_Rate : Subsystem
  Calc_climb_angle_to_SEB_rate : Subsystem
  Constant : Constant  Value=0  OutDataTypeStr=single
  Delay : Delay  DelayLength=1
  FF & Damp : Subsystem
  I : Subsystem
  Pitch_Saturation : Subsystem
  tas1 : InportShadow  Port=2
  pitch_cmd : Outport
  wires:
  ser/1 -> Calc_Seb_Rate/1(ser)
  Calc_Seb_Rate/1(seb_rate_err) -> I/1(err), FF & Damp/1(seb_rate_err)
  I/1(i_out) -> Add/2
  Delay/1 -> I/4(cmd_last), Pitch_Saturation/3(cmd_last)
  Calc_Seb_Rate/2(seb_rate_sp) -> FF & Damp/2(seb_rate_sp)
  FF & Damp/1(ff_d_out) -> Add/1
  Pitch_Saturation/1(pitch_cmd) -> pitch_cmd/1, Delay/1
  Add/1 -> Pitch_Saturation/2(ctrl_out)
  Constant/1 -> I/3(reset)
  tas/1 -> Calc_climb_angle_to_SEB_rate/1(tas)
  Calc_climb_angle_to_SEB_rate/1(climb_angle_to_SEB_rate) -> FF & Damp/3(climb_angle_to_SEB_rate), I/2(climb_angle_to_SEB_rate)
  tas1/1 -> Pitch_Saturation/1(tas)

== system Copy_of_Formation_Controller/Fixwing_Controller/Lateral_Longitudinal_Control/Longitudinal_Control/Throttle_Control ==
  note: limit
  ser : Inport
  INS_Out : Inport  Port=2
  Add : Sum
  Calc_STE_Rate : Subsystem
  Constant : Constant  Value=0  OutDataTypeStr=single
  Damp : Subsystem
  Delay : Delay  DelayLength=1
  I : Subsystem
  Saturation : Saturate  UpperLimit=CONTROL_PARAM.FW_THR_MAX  LowerLimit=CONTROL_PARAM.FW_THR_MIN
  throttle_cmd : Outport
  wires:
  ser/1 -> Calc_STE_Rate/1(ser)
  I/1(i_out) -> Add/2
  Delay/1 -> I/3(cmd_last)
  Add/1 -> Saturation/1
  Calc_STE_Rate/2(throttle_predicted) -> Damp/2(throttle_predicted)
  Saturation/1 -> throttle_cmd/1, Delay/1
  Calc_STE_Rate/1(ste_rate_err) -> Damp/1(ste_rate_err), I/1(ste_rate_err)
  Damp/1(ff_d_out) -> Add/1
  Constant/1 -> I/2(reset)
  INS_Out/1 -> Calc_STE_Rate/2(INS_Out)

== system Copy_of_Formation_Controller/Fixwing_Controller/Attitude_Control/Innerloop_Rate_Control/PI_Control/I_Control ==
  err : Inport
  reset : Inport  Port=2
  Constant : Constant  Value=[0;0;0]  OutDataTypeStr=single
  Discrete-Time Integrator : DiscreteIntegrator  ExternalReset=level  InitialConditionSource=external  SampleTime=-1  LimitOutput=on  UpperSaturationLimit=max_i  LowerSaturationLimit=min_i  ICPrevOutput=DiscIntNeverNeededParam  ICPrevScaledInput=DiscIntNeverNeededParam
  Multiply : Product  OutDataTypeStr=Inherit: Same as first input
  Mux : Mux  Inputs=3
  gain1 : Constant  Value=p_ki  OutDataTypeStr=single
  gain2 : Constant  Value=q_ki  OutDataTypeStr=single
  gain3 : Constant  Value=r_ki  OutDataTypeStr=single
  i_out : Outport  VectorParamsAs1DForOutWhenUnconnected=off
  wires:
  err/1 -> Multiply/2
  gain2/1 -> Mux/2
  gain1/1 -> Mux/1
  gain3/1 -> Mux/3
  reset/1 -> Discrete-Time Integrator/2
  Constant/1 -> Discrete-Time Integrator/3
  Discrete-Time Integrator/1 -> i_out/1
  Mux/1 -> Multiply/1
  Multiply/1 -> Discrete-Time Integrator/1

== system Copy_of_Formation_Controller/Fixwing_Controller/Attitude_Control/Innerloop_Rate_Control/PI_Control/P_Control ==
  err : Inport
  Multiply : Product  OutDataTypeStr=Inherit: Same as first input
  Mux : Mux  Inputs=3
  gain1 : Constant  Value=p_kp  OutDataTypeStr=single
  gain2 : Constant  Value=q_kp  OutDataTypeStr=single
  gain3 : Constant  Value=r_kp  OutDataTypeStr=single
  p_out : Outport  VectorParamsAs1DForOutWhenUnconnected=off
  wires:
  err/1 -> Multiply/2
  gain2/1 -> Mux/2
  Mux/1 -> Multiply/1
  gain1/1 -> Mux/1
  Multiply/1 -> p_out/1
  gain3/1 -> Mux/3

== system Copy_of_Formation_Controller/Fixwing_Controller/Attitude_Control/Outloop_Angle_Control/Attitude_Controller/Error ==
  att_cmd : Inport
  INS_Out : Inport  Port=2
  Bus_Select : Subsystem
  Demux : Demux  Outputs=2
  Mux : Mux  Inputs=2
  Pitch Offset : Bias  Bias=CONTROL_PARAM.FW_PSP_OFF  SaturateOnIntegerOverflow=off
  Sum : Sum  Inputs=|+-
  euler_err_rad : Outport  VectorParamsAs1DForOutWhenUnconnected=off
  wires:
  att_cmd/1 -> Demux/1  "att_cmd_B_rad"
  Sum/1 -> euler_err_rad/1  "att_error_B_rad"
  INS_Out/1 -> Bus_Select/1(INS_Out)
  Bus_Select/1(att_est_B_rad) -> Sum/2  "att_est_B_rad"
  Demux/2 -> Pitch Offset/1
  Demux/1 -> Mux/1
  Pitch Offset/1 -> Mux/2
  Mux/1 -> Sum/1

== system Copy_of_Formation_Controller/Fixwing_Controller/Attitude_Control/Outloop_Angle_Control/Attitude_Controller/P_Controller ==
  error : Inport
  Constant1 : Constant  Value=CONTROL_PARAM.ROLL_P
  Constant2 : Constant  Value=CONTROL_PARAM.PITCH_P
  Multiply : Product
  Mux : Mux  Inputs=2
  u : Outport  VectorParamsAs1DForOutWhenUnconnected=off
  wires:
  Multiply/1 -> u/1
  error/1 -> Multiply/1
  Mux/1 -> Multiply/2
  Constant1/1 -> Mux/1
  Constant2/1 -> Mux/2

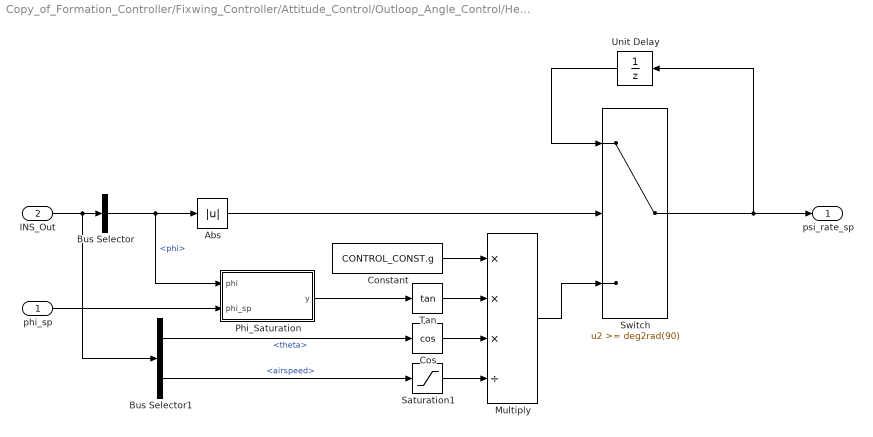
== system Copy_of_Formation_Controller/Fixwing_Controller/Attitude_Control/Outloop_Angle_Control/Heading_Controller/Turning_Coordination ==
  phi_sp : Inport
  INS_Out : Inport  Port=2
  Abs : Abs  SaturateOnIntegerOverflow=off
  Bus Selector : BusSelector  OutputSignals=phi
  Bus Selector1 : BusSelector  OutputSignals=theta,airspeed
  Constant : Constant  Value=CONTROL_CONST.g  OutDataTypeStr=single
  Cos : Trigonometry  Operator=cos
  Multiply : Product  Inputs=***/
  Phi_Saturation : Subsystem
  Saturation1 : Saturate  UpperLimit=CONTROL_PARAM.FW_AIRSPD_MAX  LowerLimit=CONTROL_PARAM.FW_AIRSPD_STALL
  Switch : Switch  Threshold=deg2rad(90)  SaturateOnIntegerOverflow=off  InputSameDT=off
  Tan : Trigonometry  Operator=tan
  Unit Delay : UnitDelay  SampleTime=-1  HasFrameUpgradeWarning=on
  psi_rate_sp : Outport  VectorParamsAs1DForOutWhenUnconnected=off
  wires:
  Tan/1 -> Multiply/2
  Cos/1 -> Multiply/3
  Bus Selector/1 -> Phi_Saturation/1(phi), Abs/1  "<phi>"
  INS_Out/1 -> Bus Selector/1, Bus Selector1/1
  Bus Selector1/1 -> Cos/1  "<theta>"
  Abs/1 -> Switch/2
  Unit Delay/1 -> Switch/1
  Multiply/1 -> Switch/3
  Switch/1 -> Unit Delay/1, psi_rate_sp/1
  Constant/1 -> Multiply/1
  Saturation1/1 -> Multiply/4
  Bus Selector1/2 -> Saturation1/1  "<airspeed>"
  phi_sp/1 -> Phi_Saturation/2(phi_sp)
  Phi_Saturation/1(y) -> Tan/1

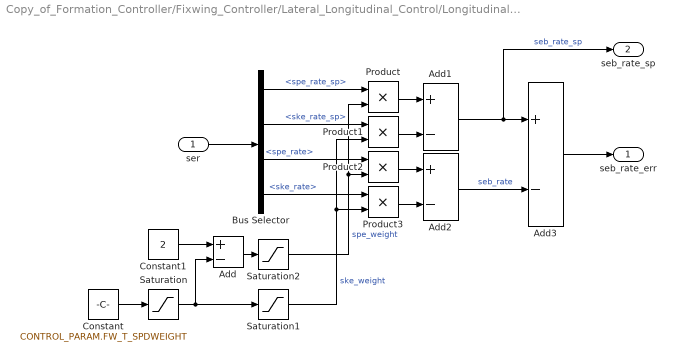
== system Copy_of_Formation_Controller/Fixwing_Controller/Lateral_Longitudinal_Control/Longitudinal_Control/Pitch_Control/Calc_Seb_Rate ==
  ser : Inport
  Add{,1..3} (4 alike) : Sum  Inputs=+-
  Bus Selector : BusSelector  OutputSignals=spe_rate_sp,ske_rate_sp,spe_rate,ske_rate
  Constant : Constant  Value=CONTROL_PARAM.FW_T_SPDWEIGHT  OutDataTypeStr=single
  Constant1 : Constant  Value=2  OutDataTypeStr=single
  Product{,1..3} (4 alike) : Product
  Saturation : Saturate  UpperLimit=2  LowerLimit=0
  Saturation1 : Saturate  UpperLimit=1  LowerLimit=0
  Saturation2 : Saturate  UpperLimit=1  LowerLimit=0
  seb_rate_err : Outport
  seb_rate_sp : Outport  Port=2
  wires:
  Saturation2/1 -> Product2/2, Product/2  "spe_weight"
  Add/1 -> Saturation2/1
  Saturation/1 -> Add/2, Saturation1/1
  Saturation1/1 -> Product1/2, Product3/2  "ske_weight"
  Constant1/1 -> Add/1
  Constant/1 -> Saturation/1
  ser/1 -> Bus Selector/1
  Bus Selector/1 -> Product/1  "<spe_rate_sp>"
  Bus Selector/2 -> Product1/1  "<ske_rate_sp>"
  Bus Selector/3 -> Product2/1  "<spe_rate>"
  Bus Selector/4 -> Product3/1  "<ske_rate>"
  Product1/1 -> Add1/2
  Product/1 -> Add1/1
  Product2/1 -> Add2/1
  Product3/1 -> Add2/2
  Add1/1 -> seb_rate_sp/1, Add3/1  "seb_rate_sp"
  Add2/1 -> Add3/2  "seb_rate"
  Add3/1 -> seb_rate_err/1

== system Copy_of_Formation_Controller/Fixwing_Controller/Lateral_Longitudinal_Control/Longitudinal_Control/Pitch_Control/Calc_climb_angle_to_SEB_rate ==
  tas : Inport
  Constant1 : Constant  Value=CONTROL_CONST.g
  Product : Product
  climb_angle_to_SEB_rate : Outport
  wires:
  Constant1/1 -> Product/1
  Product/1 -> climb_angle_to_SEB_rate/1
  tas/1 -> Product/2

== system Copy_of_Formation_Controller/Fixwing_Controller/Lateral_Longitudinal_Control/Longitudinal_Control/Pitch_Control/FF & Damp ==
  seb_rate_err : Inport
  seb_rate_sp : Inport  Port=2
  climb_angle_to_SEB_rate : Inport  Port=3
  Add : Sum
  Divide : Product  Inputs=*/
  pitch_damping_gain : Gain  Gain=CONTROL_PARAM.FW_T_PTCH_DAMP
  seb_rate_ff : Gain  Gain=CONTROL_PARAM.FW_T_SEB_R_FF
  ff_d_out : Outport
  wires:
  seb_rate_err/1 -> pitch_damping_gain/1
  seb_rate_sp/1 -> seb_rate_ff/1
  pitch_damping_gain/1 -> Add/1
  seb_rate_ff/1 -> Add/2
  Add/1 -> Divide/1
  climb_angle_to_SEB_rate/1 -> Divide/2
  Divide/1 -> ff_d_out/1

== system Copy_of_Formation_Controller/Fixwing_Controller/Lateral_Longitudinal_Control/Longitudinal_Control/Pitch_Control/I ==
  err : Inport
  climb_angle_to_SEB_rate : Inport  Port=2
  reset : Inport  Port=3
  cmd_last : Inport  Port=4
  Discrete-Time Integrator : DiscreteIntegrator  gainval=1  ExternalReset=level  SampleTime=-1  ICPrevOutput=DiscIntNeverNeededParam  ICPrevScaledInput=DiscIntNeverNeededParam
  Divide : Product  Inputs=*/
  Error_Saturation : MATLAB Function  TreatAsAtomicUnit=on  mask{uplimit=CONTROL_PARAM.FW_P_LIM_MAX, downlimit=CONTROL_PARAM.FW_P_LIM_MIN}
      mask prompts: uplimit "MaxOutput"; downlimit "MinOutput"
  I_Gain : Gain  Gain=CONTROL_PARAM.FW_T_I_GAIN_PIT
  i_out : Outport
  wires:
  Discrete-Time Integrator/1 -> i_out/1
  err/1 -> Divide/1
  cmd_last/1 -> Error_Saturation/2(cmd_last)
  Error_Saturation/1(y) -> I_Gain/1
  reset/1 -> Discrete-Time Integrator/2
  climb_angle_to_SEB_rate/1 -> Divide/2
  Divide/1 -> Error_Saturation/1(err)
  I_Gain/1 -> Discrete-Time Integrator/1

== system Copy_of_Formation_Controller/Fixwing_Controller/Lateral_Longitudinal_Control/Longitudinal_Control/Pitch_Control/Pitch_Saturation ==
  note: saturation
  tas : Inport
  ctrl_out : Inport  Port=2
  cmd_last : Inport  Port=3
  Pitch_Saturation : MATLAB Function  Commented=on  TreatAsAtomicUnit=on  mask{dt=CONTROL_CONST.dt, limit=CONTROL_PARAM.FW_T_VERT_ACC}
      mask prompts: limit "vert_accel_limit"
  Saturation : Saturate  UpperLimit=CONTROL_PARAM.FW_P_LIM_MAX  LowerLimit=CONTROL_PARAM.FW_P_LIM_MIN
  pitch_cmd : Outport
  wires:
  ctrl_out/1 -> Saturation/1
  cmd_last/1 -> Pitch_Saturation/3(y_last)
  Saturation/1 -> pitch_cmd/1, Pitch_Saturation/1(u)
  tas/1 -> Pitch_Saturation/2(tas)

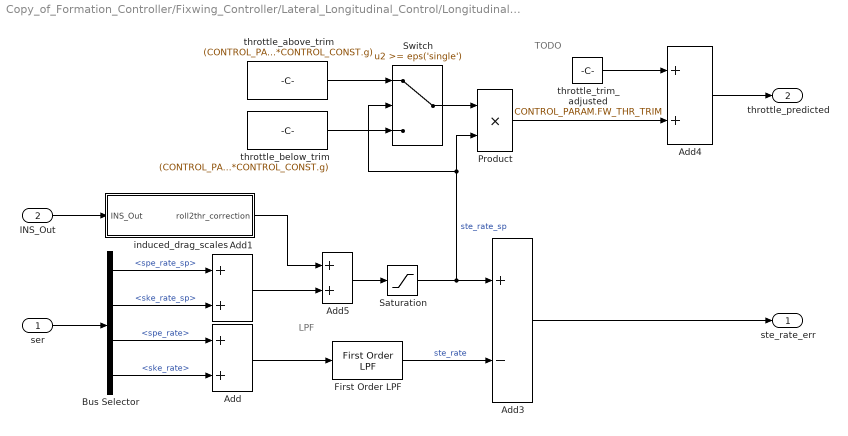
== system Copy_of_Formation_Controller/Fixwing_Controller/Lateral_Longitudinal_Control/Longitudinal_Control/Throttle_Control/Calc_STE_Rate ==
  note: TODO
  note: LPF
  ser : Inport
  INS_Out : Inport  Port=2
  Add{,1,4..5} (4 alike) : Sum
  Add3 : Sum  Inputs=+-
  Bus Selector : BusSelector  OutputSignals=spe_rate_sp,ske_rate_sp,spe_rate,ske_rate
  First Order LPF : FC_Lib/Filter/First Order LPF  fc=1/(2*pi*0.4)
      settings: SourceProductName=Flight Control Toolbox
  Product : Product
  Saturation : Saturate  UpperLimit=CONTROL_PARAM.FW_T_CLMB_MAX*CONTROL_CONST.g  LowerLimit=-CONTROL_PARAM.FW_T_SINK_MIN*CONTROL_CONST.g
  Switch : Switch  Threshold=eps('single')  SaturateOnIntegerOverflow=off  InputSameDT=off
  induced_drag_scales : Subsystem
  throttle_above_trim : Constant  Value=(CONTROL_PARAM.FW_THR_MAX-CONTROL_PARAM.FW_THR_TRIM)/(CONTROL_PARAM.FW_T_CLMB_MAX*CONTROL_CONST.g)
  throttle_below_trim : Constant  Value=(CONTROL_PARAM.FW_THR_TRIM-CONTROL_PARAM.FW_THR_MIN)/(CONTROL_PARAM.FW_T_SINK_MIN*CONTROL_CONST.g)
  throttle_trim_adjusted : Constant  Value=CONTROL_PARAM.FW_THR_TRIM  OutDataTypeStr=single
  ste_rate_err : Outport
  throttle_predicted : Outport  Port=2
  wires:
  Bus Selector/3 -> Add/1  "<spe_rate>"
  Add/1 -> First Order LPF/1
  Bus Selector/2 -> Add1/2  "<ske_rate_sp>"
  Add1/1 -> Add5/2
  Bus Selector/4 -> Add/2  "<ske_rate>"
  Bus Selector/1 -> Add1/1  "<spe_rate_sp>"
  ser/1 -> Bus Selector/1
  First Order LPF/1 -> Add3/2  "ste_rate"
  Saturation/1 -> Switch/2, Product/2, Add3/1  "ste_rate_sp"
  Add3/1 -> ste_rate_err/1
  throttle_below_trim/1 -> Switch/3
  throttle_above_trim/1 -> Switch/1
  Switch/1 -> Product/1
  throttle_trim_adjusted/1 -> Add4/1
  Product/1 -> Add4/2
  Add4/1 -> throttle_predicted/1
  Add5/1 -> Saturation/1
  INS_Out/1 -> induced_drag_scales/1(INS_Out)
  induced_drag_scales/1(roll2thr_correction) -> Add5/1

== system Copy_of_Formation_Controller/Fixwing_Controller/Lateral_Longitudinal_Control/Longitudinal_Control/Throttle_Control/Damp ==
  ste_rate_err : Inport
  throttle_predicted : Inport  Port=2
  Add : Sum
  Product : Product
  STE_rate_to_throttle : Constant  Value=CONTROL_CONST.g*(CONTROL_PARAM.FW_T_CLMB_MAX+CONTROL_PARAM.FW_T_SINK_MAX)
  throttle_damping_gain : Gain  Gain=CONTROL_PARAM.FW_T_THR_DAMP
  ff_d_out : Outport
  wires:
  ste_rate_err/1 -> throttle_damping_gain/1
  throttle_damping_gain/1 -> Product/1
  throttle_predicted/1 -> Add/2
  Add/1 -> ff_d_out/1
  Product/1 -> Add/1
  STE_rate_to_throttle/1 -> Product/2

== system Copy_of_Formation_Controller/Fixwing_Controller/Lateral_Longitudinal_Control/Longitudinal_Control/Throttle_Control/I ==
  ste_rate_err : Inport
  reset : Inport  Port=2
  cmd_last : Inport  Port=3
  Discrete-Time Integrator : DiscreteIntegrator  gainval=1  ExternalReset=level  SampleTime=-1  ICPrevOutput=DiscIntNeverNeededParam  ICPrevScaledInput=DiscIntNeverNeededParam
  Error_Saturation : MATLAB Function  TreatAsAtomicUnit=on  mask{uplimit=CONTROL_PARAM.FW_THR_MAX, downlimit=CONTROL_PARAM.FW_THR_MIN}
      mask prompts: uplimit "MaxOutput"; downlimit "MinOutput"
  I_Gain : Gain  Gain=CONTROL_PARAM.FW_T_I_GAIN_THR
  Product : Product
  STE_rate_to_throttle : Constant  Value=CONTROL_CONST.g*(CONTROL_PARAM.FW_T_CLMB_MAX+CONTROL_PARAM.FW_T_SINK_MAX)
  i_out : Outport
  wires:
  Discrete-Time Integrator/1 -> i_out/1
  cmd_last/1 -> Error_Saturation/2(cmd_last)
  ste_rate_err/1 -> Product/1
  STE_rate_to_throttle/1 -> Product/2
  Error_Saturation/1(y) -> I_Gain/1
  Product/1 -> Error_Saturation/1(err)
  reset/1 -> Discrete-Time Integrator/2
  I_Gain/1 -> Discrete-Time Integrator/1

== system Copy_of_Formation_Controller/Fixwing_Controller/Attitude_Control/Outloop_Angle_Control/Attitude_Controller/Error/Bus_Select ==
  INS_Out : Inport
  Bus Selector1 : BusSelector  OutputSignals=phi,theta
  Mux1 : Mux  Inputs=2
  att_est_B_rad : Outport  VectorParamsAs1DForOutWhenUnconnected=off
  wires:
  Bus Selector1/2 -> Mux1/2  "<theta>"
  Bus Selector1/1 -> Mux1/1  "<phi>"
  Mux1/1 -> att_est_B_rad/1
  INS_Out/1 -> Bus Selector1/1

== system Copy_of_Formation_Controller/Fixwing_Controller/Attitude_Control/Outloop_Angle_Control/Heading_Controller/Turning_Coordination/Phi_Saturation ==
  phi : Inport
  phi_sp : Inport  Port=2
  Abs1 : Abs  SaturateOnIntegerOverflow=off
  Gain : Gain  Gain=-1
  Saturation Dynamic : simulink/Discontinuities/Saturation Dynamic  OutMin=[]  OutMax=[]  OutDataTypeStr=Inherit: Same as second input  OutDataType=fixdt(1, 16)  OutScaling=2^-10  DoSatur=off
  Saturation2 : Saturate  UpperLimit=deg2rad(80)  LowerLimit=-deg2rad(80)
  y : Outport
  wires:
  Gain/1 -> Saturation Dynamic/3
  Abs1/1 -> Gain/1, Saturation Dynamic/1
  phi/1 -> Saturation2/1
  phi_sp/1 -> Abs1/1
  Saturation2/1 -> Saturation Dynamic/2
  Saturation Dynamic/1 -> y/1

== system Copy_of_Formation_Controller/Fixwing_Controller/Lateral_Longitudinal_Control/Longitudinal_Control/Throttle_Control/Calc_STE_Rate/induced_drag_scales ==
  INS_Out : Inport
  Bias : Bias  Bias=-1  SaturateOnIntegerOverflow=off
  Bus Selector1 : BusSelector  OutputSignals=phi
  Constant1 : Constant  OutDataTypeStr=single
  Cos : Trigonometry  Operator=cos
  Divide3 : Product  Inputs=*/
  load_factor_correction : Gain  Gain=CONTROL_PARAM.FW_T_RLL2THR
  roll2thr_correction : Outport
  wires:
  INS_Out/1 -> Bus Selector1/1
  Bus Selector1/1 -> Cos/1  "<phi>"
  Constant1/1 -> Divide3/1
  Cos/1 -> Divide3/2
  Divide3/1 -> Bias/1
  Bias/1 -> load_factor_correction/1
  load_factor_correction/1 -> roll2thr_correction/1

== matlab function Copy_of_Formation_Controller/Fixwing_Controller/Lateral_Longitudinal_Control/Longitudinal_Control/Pitch_Control/Pitch_Saturation/Pitch_Saturation ==
  data: u input; tas input; y output; limit parameter; dt parameter; y_last input
function y = fcn(u, tas, limit, dt, y_last)
pitch_increment = dt * limit / max(tas, eps('single'));
u_min = y_last - pitch_increment;
u_max = y_last + pitch_increment;

if u < u_min
    y = u_min;
else 
    if u > u_max
        y = u_max;
    else
        y = u;
    end
end

== matlab function Copy_of_Formation_Controller/Fixwing_Controller/Lateral_Longitudinal_Control/Longitudinal_Control/Throttle_Control/I/Error_Saturation ==
  data: err input; cmd_last input; y output; uplimit parameter; downlimit parameter
function y = fcn(err, cmd_last, uplimit, downlimit)

if cmd_last >= uplimit
    y = min(err, 0);
elseif cmd_last <= downlimit
    y = max(err, 0);
else
    y = err;
end
end

== matlab function Copy_of_Formation_Controller/Fixwing_Controller/Lateral_Longitudinal_Control/Altitude_Control/Calc_Height_Rate_Setpoint/signNoZero ==
  data: u input; y output
function y = fcn(u)

y = cast((0 <= u) - (u < 0), 'like', u);

== matlab function Copy_of_Formation_Controller/Fixwing_Controller/Lateral_Longitudinal_Control/Altitude_Control/Calc_Height_Rate_Setpoint/computeMaxSpeedFromDistance ==
  data: jerk input; max_speed output; accel input; braking_distance input; final_speed input
function max_speed = fcn(jerk, accel, braking_distance, final_speed)
    sqr = @(f) f * f;
    b = 4.0 * sqr(accel) / jerk;
    c = -2.0 * accel * braking_distance - sqr(final_speed);
    max_speed = 0.5 * (-b + sqrt(sqr(b) - 4.0 * c));
    
    % 不要减速超过最终速度，即使保守的加速度请求时间要求减速更多
    max_speed = max(max_speed, final_speed);
end

== matlab function Copy_of_Formation_Controller/Fixwing_Controller/Lateral_Longitudinal_Control/Longitudinal_Control/Pitch_Control/I/Error_Saturation ==
  data: err input; cmd_last input; y output; uplimit parameter; downlimit parameter
function y = fcn(err, cmd_last, uplimit, downlimit)

if cmd_last >= uplimit
    y = min(err, 0);
elseif cmd_last <= downlimit
    y = max(err, 0);
else
    y = err;
end
end
